simulink subsystem "RackAndPinion"  (R2023a)
settings: Solver=VariableStepAuto  StartTime=0.0  StopTime=10.0  RelTol=1e-3
model mask{i_gear=20, J_gear=1, Friction_coeff_gear=0.001}
  mask prompts: i_gear "Gear coefficient (rad/mm)"; J_gear "Gear inertia (kg*mm^2)"; Friction_coeff_gear "Friction coefficient"
settings Model: Creator=user  LastModifiedBy=user

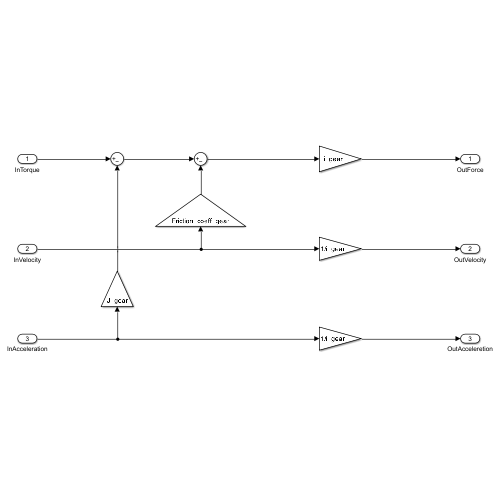
[thumbnail: Simulink's stored preview of the top-level diagram]
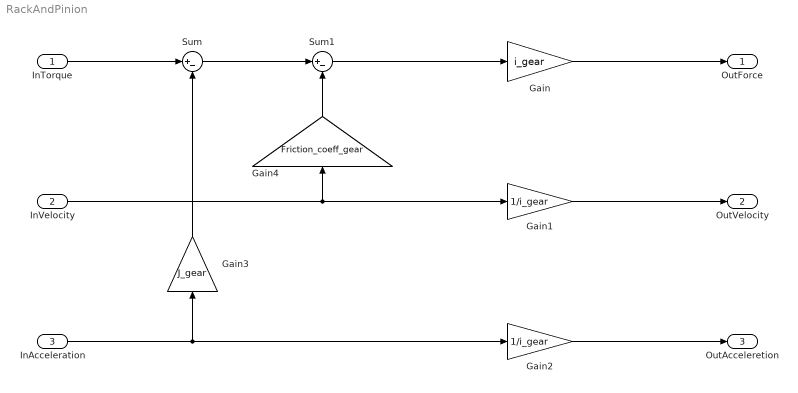
== system RackAndPinion ==
  InTorque : Inport
  InVelocity : Inport  Port=2
  InAcceleration : Inport  Port=3
  Gain : Gain  Gain=i_gear
  Gain1 : Gain  Gain=1/i_gear
  Gain2 : Gain  Gain=1/i_gear
  Gain3 : Gain  Gain=J_gear
  Gain4 : Gain  Gain=Friction_coeff_gear
  Sum : Sum  Inputs=|+-
  Sum1 : Sum  Inputs=|+-
  OutForce : Outport
  OutVelocity : Outport  Port=2
  OutAcceleretion : Outport  Port=3
  wires:
  Sum/1 -> Sum1/1
  Gain3/1 -> Sum/2
  Sum1/1 -> Gain/1
  Gain4/1 -> Sum1/2
  Gain/1 -> OutForce/1
  Gain1/1 -> OutVelocity/1
  Gain2/1 -> OutAcceleretion/1
  InTorque/1 -> Sum/1
  InAcceleration/1 -> Gain2/1, Gain3/1
  InVelocity/1 -> Gain4/1, Gain1/1
